simulink model "pasp_16i16c128s"  (Simulink 6.2)
settings: Solver=ode45  StartTime=0.0  StopTime=30000  RelTol=1e-3
undefined symbols (not defined in the file or in its folder): iBOB
libraries: xbsIndex_r3 x1501, casper_library x145, xps_library x90
(part 3 of 12)

== system pasp_16i16c128s/pasp/pfb_fir_real1 ==
  sync : Inport  Port=1  LatchInput=off
  pol1_in1 : Inport  Port=2  LatchInput=off
  pol1_in2 : Inport  Port=3  LatchInput=off
  pol1_in3 : Inport  Port=4  LatchInput=off
  pol1_in4 : Inport  Port=5  LatchInput=off
  pol1_in1_first_tap : Subsystem  AncestorBlock=casper_library/PFBs/first_tap_real  mask(first_tap_real){nput=0, PFBSize=5, CoeffBitWidth=8, TotalTaps=2, BitWidthIn=8, CoeffDistMem=1, CoeffRound=0, WindowType=hamming, mult_latency=2, bram_latency=2, n_inputs=2, fwidth=1}
      mask prompts: nput "This is input number:"; PFBSize "Size of PFB: (2^? pnts)"; CoeffBitWidth "Bitwidth of Coefficients:"; TotalTaps "Total Number of Taps:"; BitWidthIn "Input Bitwidth:"; CoeffDistMem "Implement Coeff Gen in Distributed Memory:"; CoeffRound "Round Coefficients?"; WindowType "Windowing Function:"; mult_latency "Mult Latency"; bram_latency "BRAM Latency"; n_inputs "Number of Simultaneous Inputs: (2^?)"; fwidth "Bit Width (normal=1)"
      mask init: same as pasp_16i16c128s/pasp/pfb_fir_real/pol1_in1_first_tap
      settings: AttributesFormatString=input=0, taps=2
      mask StyleString: edit,edit,edit,edit,edit,edit,edit,popup(bartlett|barthannwin|blackman|blackmanharris|bohamwin|chebwin|flattopwin|gausswin|hamming|hann|kaiser|nuttallwin|parzenwin|rectwin|tukeywin|triang),edit,edit,edit,edit
  pol1_in1_last_tap : Subsystem  AncestorBlock=casper_library/PFBs/last_tap_real  mask(last_tap_real){TotalTaps=2, BitWidthIn=8, BitWidthOut=18, CoeffBitWidth=8, add_latency=1, mult_latency=2, quantization=Truncate}
      mask prompts: TotalTaps "Total Number of Taps:"; BitWidthIn "Input Bitwidth:"; BitWidthOut "Output Bitwidth:"; CoeffBitWidth "Coeff Bitwidth:"; add_latency "Add Latency"; mult_latency "Mult Latency"; quantization "Quantization Behavior"
      mask init: same as pasp_16i16c128s/pasp/pfb_fir_real/pol1_in1_last_tap
      settings: AttributesFormatString=taps=2
      mask StyleString: edit,edit,edit,edit,edit,edit,popup(Truncate|Round  (unbiased: +/- Inf)|Round  (unbiased: Even Values))
  pol1_in2_first_tap : Subsystem  AncestorBlock=casper_library/PFBs/first_tap_real  mask(first_tap_real){nput=1, PFBSize=5, CoeffBitWidth=8, TotalTaps=2, BitWidthIn=8, CoeffDistMem=1, CoeffRound=0, WindowType=hamming, mult_latency=2, bram_latency=2, n_inputs=2, fwidth=1}
      mask prompts: nput "This is input number:"; PFBSize "Size of PFB: (2^? pnts)"; CoeffBitWidth "Bitwidth of Coefficients:"; TotalTaps "Total Number of Taps:"; BitWidthIn "Input Bitwidth:"; CoeffDistMem "Implement Coeff Gen in Distributed Memory:"; CoeffRound "Round Coefficients?"; WindowType "Windowing Function:"; mult_latency "Mult Latency"; bram_latency "BRAM Latency"; n_inputs "Number of Simultaneous Inputs: (2^?)"; fwidth "Bit Width (normal=1)"
      mask init: same as pasp_16i16c128s/pasp/pfb_fir_real/pol1_in1_first_tap
      settings: AttributesFormatString=input=1, taps=2
      mask StyleString: edit,edit,edit,edit,edit,edit,edit,popup(bartlett|barthannwin|blackman|blackmanharris|bohamwin|chebwin|flattopwin|gausswin|hamming|hann|kaiser|nuttallwin|parzenwin|rectwin|tukeywin|triang),edit,edit,edit,edit
  pol1_in2_last_tap : Subsystem  AncestorBlock=casper_library/PFBs/last_tap_real  mask(last_tap_real){TotalTaps=2, BitWidthIn=8, BitWidthOut=18, CoeffBitWidth=8, add_latency=1, mult_latency=2, quantization=Truncate}
      mask prompts: TotalTaps "Total Number of Taps:"; BitWidthIn "Input Bitwidth:"; BitWidthOut "Output Bitwidth:"; CoeffBitWidth "Coeff Bitwidth:"; add_latency "Add Latency"; mult_latency "Mult Latency"; quantization "Quantization Behavior"
      mask init: same as pasp_16i16c128s/pasp/pfb_fir_real/pol1_in1_last_tap
      settings: AttributesFormatString=taps=2
      mask StyleString: edit,edit,edit,edit,edit,edit,popup(Truncate|Round  (unbiased: +/- Inf)|Round  (unbiased: Even Values))
  pol1_in3_first_tap : Subsystem  AncestorBlock=casper_library/PFBs/first_tap_real  mask(first_tap_real){nput=2, PFBSize=5, CoeffBitWidth=8, TotalTaps=2, BitWidthIn=8, CoeffDistMem=1, CoeffRound=0, WindowType=hamming, mult_latency=2, bram_latency=2, n_inputs=2, fwidth=1}
      mask prompts: nput "This is input number:"; PFBSize "Size of PFB: (2^? pnts)"; CoeffBitWidth "Bitwidth of Coefficients:"; TotalTaps "Total Number of Taps:"; BitWidthIn "Input Bitwidth:"; CoeffDistMem "Implement Coeff Gen in Distributed Memory:"; CoeffRound "Round Coefficients?"; WindowType "Windowing Function:"; mult_latency "Mult Latency"; bram_latency "BRAM Latency"; n_inputs "Number of Simultaneous Inputs: (2^?)"; fwidth "Bit Width (normal=1)"
      mask init: same as pasp_16i16c128s/pasp/pfb_fir_real/pol1_in1_first_tap
      settings: AttributesFormatString=input=2, taps=2
      mask StyleString: edit,edit,edit,edit,edit,edit,edit,popup(bartlett|barthannwin|blackman|blackmanharris|bohamwin|chebwin|flattopwin|gausswin|hamming|hann|kaiser|nuttallwin|parzenwin|rectwin|tukeywin|triang),edit,edit,edit,edit
  pol1_in3_last_tap : Subsystem  AncestorBlock=casper_library/PFBs/last_tap_real  mask(last_tap_real){TotalTaps=2, BitWidthIn=8, BitWidthOut=18, CoeffBitWidth=8, add_latency=1, mult_latency=2, quantization=Truncate}
      mask prompts: TotalTaps "Total Number of Taps:"; BitWidthIn "Input Bitwidth:"; BitWidthOut "Output Bitwidth:"; CoeffBitWidth "Coeff Bitwidth:"; add_latency "Add Latency"; mult_latency "Mult Latency"; quantization "Quantization Behavior"
      mask init: same as pasp_16i16c128s/pasp/pfb_fir_real/pol1_in1_last_tap
      settings: AttributesFormatString=taps=2
      mask StyleString: edit,edit,edit,edit,edit,edit,popup(Truncate|Round  (unbiased: +/- Inf)|Round  (unbiased: Even Values))
  pol1_in4_first_tap : Subsystem  AncestorBlock=casper_library/PFBs/first_tap_real  mask(first_tap_real){nput=3, PFBSize=5, CoeffBitWidth=8, TotalTaps=2, BitWidthIn=8, CoeffDistMem=1, CoeffRound=0, WindowType=hamming, mult_latency=2, bram_latency=2, n_inputs=2, fwidth=1}
      mask prompts: nput "This is input number:"; PFBSize "Size of PFB: (2^? pnts)"; CoeffBitWidth "Bitwidth of Coefficients:"; TotalTaps "Total Number of Taps:"; BitWidthIn "Input Bitwidth:"; CoeffDistMem "Implement Coeff Gen in Distributed Memory:"; CoeffRound "Round Coefficients?"; WindowType "Windowing Function:"; mult_latency "Mult Latency"; bram_latency "BRAM Latency"; n_inputs "Number of Simultaneous Inputs: (2^?)"; fwidth "Bit Width (normal=1)"
      mask init: same as pasp_16i16c128s/pasp/pfb_fir_real/pol1_in1_first_tap
      settings: AttributesFormatString=input=3, taps=2
      mask StyleString: edit,edit,edit,edit,edit,edit,edit,popup(bartlett|barthannwin|blackman|blackmanharris|bohamwin|chebwin|flattopwin|gausswin|hamming|hann|kaiser|nuttallwin|parzenwin|rectwin|tukeywin|triang),edit,edit,edit,edit
  pol1_in4_last_tap : Subsystem  AncestorBlock=casper_library/PFBs/last_tap_real  mask(last_tap_real){TotalTaps=2, BitWidthIn=8, BitWidthOut=18, CoeffBitWidth=8, add_latency=1, mult_latency=2, quantization=Truncate}
      mask prompts: TotalTaps "Total Number of Taps:"; BitWidthIn "Input Bitwidth:"; BitWidthOut "Output Bitwidth:"; CoeffBitWidth "Coeff Bitwidth:"; add_latency "Add Latency"; mult_latency "Mult Latency"; quantization "Quantization Behavior"
      mask init: same as pasp_16i16c128s/pasp/pfb_fir_real/pol1_in1_last_tap
      settings: AttributesFormatString=taps=2
      mask StyleString: edit,edit,edit,edit,edit,edit,popup(Truncate|Round  (unbiased: +/- Inf)|Round  (unbiased: Even Values))
  sync_out : Outport
  pol1_out1 : Outport  Port=2
  pol1_out2 : Outport  Port=3
  pol1_out3 : Outport  Port=4
  pol1_out4 : Outport  Port=5
  wires:
  pol1_in1/1 -> pol1_in1_first_tap/1(din)
  sync/1 -> pol1_in1_first_tap/2(sync), pol1_in2_first_tap/2(sync), pol1_in3_first_tap/2(sync), pol1_in4_first_tap/2(sync)
  pol1_in1_first_tap/1(dout) -> pol1_in1_last_tap/1(din)
  pol1_in1_first_tap/2(sync_out) -> pol1_in1_last_tap/2(sync)
  pol1_in1_first_tap/3(coeff_out) -> pol1_in1_last_tap/3(coeff)
  pol1_in1_first_tap/4(taps_out) -> pol1_in1_last_tap/4(taps)
  pol1_in1_last_tap/1(dout) -> pol1_out1/1
  pol1_in1_last_tap/2(sync_out) -> sync_out/1
  pol1_in2/1 -> pol1_in2_first_tap/1(din)
  pol1_in2_first_tap/1(dout) -> pol1_in2_last_tap/1(din)
  pol1_in2_first_tap/2(sync_out) -> pol1_in2_last_tap/2(sync)
  pol1_in2_first_tap/3(coeff_out) -> pol1_in2_last_tap/3(coeff)
  pol1_in2_first_tap/4(taps_out) -> pol1_in2_last_tap/4(taps)
  pol1_in2_last_tap/1(dout) -> pol1_out2/1
  pol1_in3/1 -> pol1_in3_first_tap/1(din)
  pol1_in3_first_tap/1(dout) -> pol1_in3_last_tap/1(din)
  pol1_in3_first_tap/2(sync_out) -> pol1_in3_last_tap/2(sync)
  pol1_in3_first_tap/3(coeff_out) -> pol1_in3_last_tap/3(coeff)
  pol1_in3_first_tap/4(taps_out) -> pol1_in3_last_tap/4(taps)
  pol1_in3_last_tap/1(dout) -> pol1_out3/1
  pol1_in4/1 -> pol1_in4_first_tap/1(din)
  pol1_in4_first_tap/1(dout) -> pol1_in4_last_tap/1(din)
  pol1_in4_first_tap/2(sync_out) -> pol1_in4_last_tap/2(sync)
  pol1_in4_first_tap/3(coeff_out) -> pol1_in4_last_tap/3(coeff)
  pol1_in4_first_tap/4(taps_out) -> pol1_in4_last_tap/4(taps)
  pol1_in4_last_tap/1(dout) -> pol1_out4/1

== system pasp_16i16c128s/pasp/reorder ==
  sync : Inport  Port=1  LatchInput=off
  en : Inport  Port=2  LatchInput=off
  din0 : Inport  Port=3  LatchInput=off
  din1 : Inport  Port=4  LatchInput=off
  Counter : xbsIndex_r3/Counter  cnt_type=Count Limited  n_bits=6  bin_pt=0  arith_type=Unsigned  start_count=0  cnt_to=63  cnt_by_val=1  operation=Up  explicit_period=off  period=1  load_pin=off  rst=on  en=on  dbl_ovrd=off  show_param=off  use_rpm=on  gen_core=off
      settings: xl_area=[0, 0, 0, 0, 0, 0, 0]
  Mux : xbsIndex_r3/Mux  inputs=4  precision=Full  arith_type="Signed  (2's comp)"  n_bits=8  bin_pt=2  quantization=Truncate  overflow=Wrap  latency=1  explicit_period=off  period=1  en=off  dbl_ovrd=off  show_param=off  mux_type=off  use_rpm=off  gen_core=off
      settings: xl_area=[0, 0, 0, 0, 0, 0, 0]
  Slice1 : xbsIndex_r3/Slice  mode=Upper Bit Location + Width  nbits=2  bit1=0  base1=MSB of Input  bit0=0  base0=LSB of Input  boolean_output=off  explicit_period=off  period=1  dbl_ovrd=off
  Slice2 : xbsIndex_r3/Slice  mode=Lower Bit Location + Width  nbits=4  bit1=0  base1=MSB of Input  bit0=0  base0=LSB of Input  boolean_output=off  explicit_period=off  period=1  dbl_ovrd=off
  bram0 : xbsIndex_r3/Single Port RAM  depth=16  initVector=sin(pi*(0:15)/16)  write_mode=Read Before Write  latency=2  init_zero=on  explicit_period=off  period=1  rst=off  init_reg=0  en=off  dbl_ovrd=off  show_param=off  distributed_mem=off  use_rpm=off  gen_core=off
      settings: xl_area=[0, 0, 0, 0, 0, 0, 0]
  bram1 : xbsIndex_r3/Single Port RAM  depth=16  initVector=sin(pi*(0:15)/16)  write_mode=Read Before Write  latency=2  init_zero=on  explicit_period=off  period=1  rst=off  init_reg=0  en=off  dbl_ovrd=off  show_param=off  distributed_mem=off  use_rpm=off  gen_core=off
      settings: xl_area=[0, 0, 0, 0, 0, 0, 0]
  delay_d0 : xbsIndex_r3/Delay  latency=3  reg_retiming=off  explicit_period=off  period=1  en=off  accept_only_valid=off  init_zero=on  dbl_ovrd=off  show_param=off
      settings: xl_area=[0, 0, 0, 0, 0, 0, 0]
  delay_din0 : xbsIndex_r3/Delay  latency=4  reg_retiming=off  explicit_period=off  period=1  en=off  accept_only_valid=off  init_zero=on  dbl_ovrd=off  show_param=off
      settings: xl_area=[0, 0, 0, 0, 0, 0, 0]
  delay_din1 : xbsIndex_r3/Delay  latency=4  reg_retiming=off  explicit_period=off  period=1  en=off  accept_only_valid=off  init_zero=on  dbl_ovrd=off  show_param=off
      settings: xl_area=[0, 0, 0, 0, 0, 0, 0]
  delay_map1 : xbsIndex_r3/Delay  latency=2*map_latency  reg_retiming=off  explicit_period=off  period=1  en=off  accept_only_valid=off  init_zero=on  dbl_ovrd=off  show_param=off
      settings: xl_area=[0, 0, 0, 0, 0, 0, 0]
  delay_map2 : xbsIndex_r3/Delay  latency=1*map_latency  reg_retiming=off  explicit_period=off  period=1  en=off  accept_only_valid=off  init_zero=on  dbl_ovrd=off  show_param=off
      settings: xl_area=[0, 0, 0, 0, 0, 0, 0]
  delay_map3 : xbsIndex_r3/Delay  latency=0*map_latency  reg_retiming=off  explicit_period=off  period=1  en=off  accept_only_valid=off  init_zero=on  dbl_ovrd=off  show_param=off
      settings: xl_area=[0, 0, 0, 0, 0, 0, 0]
  delay_sel : xbsIndex_r3/Delay  latency=3  reg_retiming=off  explicit_period=off  period=1  en=off  accept_only_valid=off  init_zero=on  dbl_ovrd=off  show_param=off
      settings: xl_area=[0, 0, 0, 0, 0, 0, 0]
  delay_valid : xbsIndex_r3/Delay  latency=3  reg_retiming=off  explicit_period=off  period=1  en=off  accept_only_valid=off  init_zero=on  dbl_ovrd=off  show_param=off
      settings: xl_area=[0, 0, 0, 0, 0, 0, 0]
  delay_we : xbsIndex_r3/Delay  latency=3  reg_retiming=off  explicit_period=off  period=1  en=off  accept_only_valid=off  init_zero=on  dbl_ovrd=off  show_param=off
      settings: xl_area=[0, 0, 0, 0, 0, 0, 0]
  map1 : xbsIndex_r3/ROM  depth=16  initVector=[0 8 1 9 2 10 3 11 4 12 5 13 6 14 7 15]  arith_type=Unsigned  n_bits=4  bin_pt=0  latency=1  init_zero=on  explicit_period=off  period=1  rst=off  init_reg=0  en=off  dbl_ovrd=off  show_param=on  distributed_mem=off  use_rpm=off  gen_core=off
      settings: xl_area=[0, 0, 0, 0, 0, 0, 0]
  map2 : xbsIndex_r3/ROM  depth=16  initVector=[0 8 1 9 2 10 3 11 4 12 5 13 6 14 7 15]  arith_type=Unsigned  n_bits=4  bin_pt=0  latency=1  init_zero=on  explicit_period=off  period=1  rst=off  init_reg=0  en=off  dbl_ovrd=off  show_param=on  distributed_mem=off  use_rpm=off  gen_core=off
      settings: xl_area=[0, 0, 0, 0, 0, 0, 0]
  map3 : xbsIndex_r3/ROM  depth=16  initVector=[0 8 1 9 2 10 3 11 4 12 5 13 6 14 7 15]  arith_type=Unsigned  n_bits=4  bin_pt=0  latency=1  init_zero=on  explicit_period=off  period=1  rst=off  init_reg=0  en=off  dbl_ovrd=off  show_param=on  distributed_mem=off  use_rpm=off  gen_core=off
      settings: xl_area=[0, 0, 0, 0, 0, 0, 0]
  post_sync_delay : xbsIndex_r3/Delay  latency=3  reg_retiming=off  explicit_period=off  period=1  en=off  accept_only_valid=off  init_zero=on  dbl_ovrd=off  show_param=off
      settings: xl_area=[0, 0, 0, 0, 0, 0, 0]
  pre_sync_delay : xbsIndex_r3/Delay  latency=3  reg_retiming=off  explicit_period=off  period=1  en=off  accept_only_valid=off  init_zero=on  dbl_ovrd=off  show_param=off
      settings: xl_area=[0, 0, 0, 0, 0, 0, 0]
  sync_delay_en : casper_library/Delays/sync_delay_en  DelayLen=16
      link override Constant: equ=P=C
      link override Constant1: equ=P=C
      link override Constant2: equ=P=C
      link override Constant3: equ=P=C
  sync_out : Outport
  valid : Outport  Port=2
  dout0 : Outport  Port=3
  dout1 : Outport  Port=4
  wires:
  sync/1 -> Counter/1, pre_sync_delay/1
  en/1 -> Counter/2, sync_delay_en/2, delay_we/1
  Counter/1 -> Slice1/1, Slice2/1
  Slice1/1 -> delay_sel/1
  delay_sel/1 -> Mux/1
  Slice2/1 -> delay_d0/1, map1/1
  delay_d0/1 -> Mux/2
  pre_sync_delay/1 -> sync_delay_en/1
  sync_delay_en/1 -> post_sync_delay/1
  post_sync_delay/1 -> sync_out/1
  delay_we/1 -> delay_valid/1, bram0/3, bram1/3
  delay_valid/1 -> valid/1
  Mux/1 -> bram0/1, bram1/1
  din0/1 -> delay_din0/1
  delay_din0/1 -> bram0/2
  bram0/1 -> dout0/1
  din1/1 -> delay_din1/1
  delay_din1/1 -> bram1/2
  bram1/1 -> dout1/1
  map1/1 -> delay_map1/1, map2/1
  delay_map1/1 -> Mux/3
  map2/1 -> delay_map2/1, map3/1
  delay_map2/1 -> Mux/4
  map3/1 -> delay_map3/1
  delay_map3/1 -> Mux/5

== system pasp_16i16c128s/pasp/scale1 ==
  note: Unsigned, 18-bits, b.p. at 12
  note: Output complex signed R/I 18-bits, b.p. at 17
  note: Input complex signed R/I 18-bits, b.p. at 17
  coeff : Inport  Orientation=down  Port=1  LatchInput=off
  data_in : Inport  Port=2  LatchInput=off
  c_to_ri : casper_library/Misc/c_to_ri  n_bits=18  bin_pt=17
      settings: AttributesFormatString=18_17 r/i
  mult_coeff_fft_imag : xbsIndex_r3/Mult  precision=User Defined  arith_type="Signed  (2's comp)"  n_bits=18  bin_pt=17  quantization=Truncate  overflow=Saturate  latency=6  explicit_period=off  period=1  en=off  dbl_ovrd=off  show_param=on  mult_type=Parallel  oversample=2  use_embedded=on  pipeline=on  use_rpm=on  placement_style=Rectangular Shape  gen_core=off
      settings: xl_area=[0, 0, 0, 0, 0, 0, 0]
  mult_coeff_fft_real : xbsIndex_r3/Mult  precision=User Defined  arith_type="Signed  (2's comp)"  n_bits=18  bin_pt=17  quantization=Truncate  overflow=Saturate  latency=6  explicit_period=off  period=1  en=off  dbl_ovrd=off  show_param=on  mult_type=Parallel  oversample=2  use_embedded=on  pipeline=on  use_rpm=on  placement_style=Rectangular Shape  gen_core=off
      settings: xl_area=[0, 0, 0, 0, 0, 0, 0]
  ri_to_c : casper_library/Misc/ri_to_c
  data_out : Outport
  wires:
  c_to_ri/1 -> mult_coeff_fft_real/2
  c_to_ri/2 -> mult_coeff_fft_imag/2
  mult_coeff_fft_real/1 -> ri_to_c/1
  mult_coeff_fft_imag/1 -> ri_to_c/2
  coeff/1 -> mult_coeff_fft_real/1, mult_coeff_fft_imag/1
  ri_to_c/1 -> data_out/1
  data_in/1 -> c_to_ri/1

== system pasp_16i16c128s/pasp/scale2 ==
  note: Input complex signed R/I 18-bits, b.p. at 17
  note: Output complex signed R/I 18-bits, b.p. at 17
  note: Unsigned, 18-bits, b.p. at 12
  coeff : Inport  Orientation=down  Port=1  LatchInput=off
  data_in : Inport  Port=2  LatchInput=off
  c_to_ri : casper_library/Misc/c_to_ri  n_bits=18  bin_pt=17
      settings: AttributesFormatString=18_17 r/i
  mult_coeff_fft_imag : xbsIndex_r3/Mult  precision=User Defined  arith_type="Signed  (2's comp)"  n_bits=18  bin_pt=17  quantization=Truncate  overflow=Saturate  latency=6  explicit_period=off  period=1  en=off  dbl_ovrd=off  show_param=on  mult_type=Parallel  oversample=2  use_embedded=on  pipeline=on  use_rpm=on  placement_style=Rectangular Shape  gen_core=off
      settings: xl_area=[0, 0, 0, 0, 0, 0, 0]
  mult_coeff_fft_real : xbsIndex_r3/Mult  precision=User Defined  arith_type="Signed  (2's comp)"  n_bits=18  bin_pt=17  quantization=Truncate  overflow=Saturate  latency=6  explicit_period=off  period=1  en=off  dbl_ovrd=off  show_param=on  mult_type=Parallel  oversample=2  use_embedded=on  pipeline=on  use_rpm=on  placement_style=Rectangular Shape  gen_core=off
      settings: xl_area=[0, 0, 0, 0, 0, 0, 0]
  ri_to_c : casper_library/Misc/ri_to_c
  data_out : Outport
  wires:
  data_in/1 -> c_to_ri/1
  ri_to_c/1 -> data_out/1
  coeff/1 -> mult_coeff_fft_imag/1, mult_coeff_fft_real/1
  mult_coeff_fft_imag/1 -> ri_to_c/2
  mult_coeff_fft_real/1 -> ri_to_c/1
  c_to_ri/2 -> mult_coeff_fft_imag/2
  c_to_ri/1 -> mult_coeff_fft_real/2

== system pasp_16i16c128s/pasp/scale3 ==
  note: Unsigned, 18-bits, b.p. at 12
  note: Output complex signed R/I 18-bits, b.p. at 17
  note: Input complex signed R/I 18-bits, b.p. at 17
  coeff : Inport  Orientation=down  Port=1  LatchInput=off
  data_in : Inport  Port=2  LatchInput=off
  c_to_ri : casper_library/Misc/c_to_ri  n_bits=18  bin_pt=17
      settings: AttributesFormatString=18_17 r/i
  mult_coeff_fft_imag : xbsIndex_r3/Mult  precision=User Defined  arith_type="Signed  (2's comp)"  n_bits=18  bin_pt=17  quantization=Truncate  overflow=Saturate  latency=6  explicit_period=off  period=1  en=off  dbl_ovrd=off  show_param=on  mult_type=Parallel  oversample=2  use_embedded=on  pipeline=on  use_rpm=on  placement_style=Rectangular Shape  gen_core=off
      settings: xl_area=[0, 0, 0, 0, 0, 0, 0]
  mult_coeff_fft_real : xbsIndex_r3/Mult  precision=User Defined  arith_type="Signed  (2's comp)"  n_bits=18  bin_pt=17  quantization=Truncate  overflow=Saturate  latency=6  explicit_period=off  period=1  en=off  dbl_ovrd=off  show_param=on  mult_type=Parallel  oversample=2  use_embedded=on  pipeline=on  use_rpm=on  placement_style=Rectangular Shape  gen_core=off
      settings: xl_area=[0, 0, 0, 0, 0, 0, 0]
  ri_to_c : casper_library/Misc/ri_to_c
  data_out : Outport
  wires:
  c_to_ri/1 -> mult_coeff_fft_real/2
  c_to_ri/2 -> mult_coeff_fft_imag/2
  mult_coeff_fft_real/1 -> ri_to_c/1
  mult_coeff_fft_imag/1 -> ri_to_c/2
  coeff/1 -> mult_coeff_fft_real/1, mult_coeff_fft_imag/1
  ri_to_c/1 -> data_out/1
  data_in/1 -> c_to_ri/1

== system pasp_16i16c128s/pasp/scale4 ==
  note: Input complex signed R/I 18-bits, b.p. at 17
  note: Output complex signed R/I 18-bits, b.p. at 17
  note: Unsigned, 18-bits, b.p. at 12
  coeff : Inport  Orientation=down  Port=1  LatchInput=off
  data_in : Inport  Port=2  LatchInput=off
  c_to_ri : casper_library/Misc/c_to_ri  n_bits=18  bin_pt=17
      settings: AttributesFormatString=18_17 r/i
  mult_coeff_fft_imag : xbsIndex_r3/Mult  precision=User Defined  arith_type="Signed  (2's comp)"  n_bits=18  bin_pt=17  quantization=Truncate  overflow=Saturate  latency=6  explicit_period=off  period=1  en=off  dbl_ovrd=off  show_param=on  mult_type=Parallel  oversample=2  use_embedded=on  pipeline=on  use_rpm=on  placement_style=Rectangular Shape  gen_core=off
      settings: xl_area=[0, 0, 0, 0, 0, 0, 0]
  mult_coeff_fft_real : xbsIndex_r3/Mult  precision=User Defined  arith_type="Signed  (2's comp)"  n_bits=18  bin_pt=17  quantization=Truncate  overflow=Saturate  latency=6  explicit_period=off  period=1  en=off  dbl_ovrd=off  show_param=on  mult_type=Parallel  oversample=2  use_embedded=on  pipeline=on  use_rpm=on  placement_style=Rectangular Shape  gen_core=off
      settings: xl_area=[0, 0, 0, 0, 0, 0, 0]
  ri_to_c : casper_library/Misc/ri_to_c
  data_out : Outport
  wires:
  data_in/1 -> c_to_ri/1
  ri_to_c/1 -> data_out/1
  coeff/1 -> mult_coeff_fft_imag/1, mult_coeff_fft_real/1
  mult_coeff_fft_imag/1 -> ri_to_c/2
  mult_coeff_fft_real/1 -> ri_to_c/1
  c_to_ri/2 -> mult_coeff_fft_imag/2
  c_to_ri/1 -> mult_coeff_fft_real/2

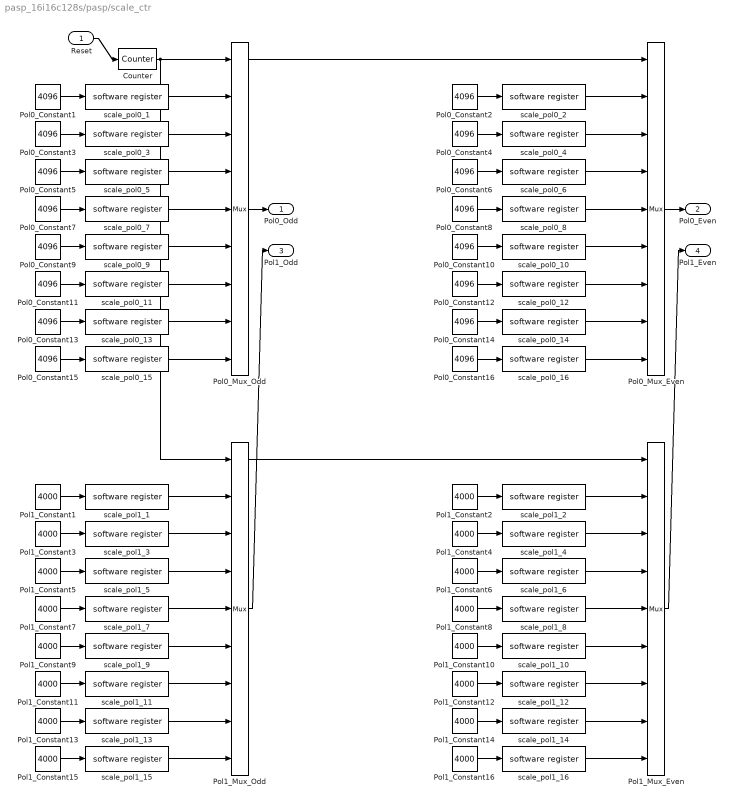
== system pasp_16i16c128s/pasp/scale_ctr ==
  Reset : Inport  Port=1  LatchInput=off
  Counter : xbsIndex_r3/Counter  cnt_type=Free Running  n_bits=3  bin_pt=0  arith_type=Unsigned  start_count=0  cnt_to=Inf  cnt_by_val=1  operation=Up  explicit_period=off  period=1  load_pin=off  rst=on  en=off  dbl_ovrd=off  show_param=off  use_rpm=on  gen_core=off
      settings: xl_area=[0, 0, 0, 0, 0, 0, 0]
  Pol0_Constant{1..16} (16 alike) : Constant  Value=4096
  Pol0_Mux_Even : xbsIndex_r3/Mux  inputs=8  precision=Full  arith_type="Signed  (2's comp)"  n_bits=8  bin_pt=2  quantization=Truncate  overflow=Wrap  latency=3  explicit_period=off  period=1  en=off  dbl_ovrd=off  show_param=off  mux_type=off  use_rpm=off  gen_core=off
      settings: xl_area=[0, 0, 0, 0, 0, 0, 0]
  Pol0_Mux_Odd : xbsIndex_r3/Mux  inputs=8  precision=Full  arith_type="Signed  (2's comp)"  n_bits=8  bin_pt=2  quantization=Truncate  overflow=Wrap  latency=3  explicit_period=off  period=1  en=off  dbl_ovrd=off  show_param=off  mux_type=off  use_rpm=off  gen_core=off
      settings: xl_area=[0, 0, 0, 0, 0, 0, 0]
  Pol1_Constant{1..16} (16 alike) : Constant  Value=4000
  Pol1_Mux_Even : xbsIndex_r3/Mux  inputs=8  precision=Full  arith_type="Signed  (2's comp)"  n_bits=8  bin_pt=2  quantization=Truncate  overflow=Wrap  latency=3  explicit_period=off  period=1  en=off  dbl_ovrd=off  show_param=off  mux_type=off  use_rpm=off  gen_core=off
      settings: xl_area=[0, 0, 0, 0, 0, 0, 0]
  Pol1_Mux_Odd : xbsIndex_r3/Mux  inputs=8  precision=Full  arith_type="Signed  (2's comp)"  n_bits=8  bin_pt=2  quantization=Truncate  overflow=Wrap  latency=3  explicit_period=off  period=1  en=off  dbl_ovrd=off  show_param=off  mux_type=off  use_rpm=off  gen_core=off
      settings: xl_area=[0, 0, 0, 0, 0, 0, 0]
  scale_pol0_1 : xps_library/software register  Tag=xps:sw_reg  io_dir=From Processor  arith_type=Unsigned  bitwidth=32  bin_pt=0  sample_period=1  gw_name=pasp_16i16c128s_pasp_scale_ctr_scale_pol0_1_user_data_out
  scale_pol0_10 : xps_library/software register  Tag=xps:sw_reg  io_dir=From Processor  arith_type=Unsigned  bitwidth=32  bin_pt=0  sample_period=1  gw_name=pasp_16i16c128s_pasp_scale_ctr_scale_pol0_10_user_data_out
  scale_pol0_11 : xps_library/software register  Tag=xps:sw_reg  io_dir=From Processor  arith_type=Unsigned  bitwidth=32  bin_pt=0  sample_period=1  gw_name=pasp_16i16c128s_pasp_scale_ctr_scale_pol0_11_user_data_out
  scale_pol0_12 : xps_library/software register  Tag=xps:sw_reg  io_dir=From Processor  arith_type=Unsigned  bitwidth=32  bin_pt=0  sample_period=1  gw_name=pasp_16i16c128s_pasp_scale_ctr_scale_pol0_12_user_data_out
  scale_pol0_13 : xps_library/software register  Tag=xps:sw_reg  io_dir=From Processor  arith_type=Unsigned  bitwidth=32  bin_pt=0  sample_period=1  gw_name=pasp_16i16c128s_pasp_scale_ctr_scale_pol0_13_user_data_out
  scale_pol0_14 : xps_library/software register  Tag=xps:sw_reg  io_dir=From Processor  arith_type=Unsigned  bitwidth=32  bin_pt=0  sample_period=1  gw_name=pasp_16i16c128s_pasp_scale_ctr_scale_pol0_14_user_data_out
  scale_pol0_15 : xps_library/software register  Tag=xps:sw_reg  io_dir=From Processor  arith_type=Unsigned  bitwidth=32  bin_pt=0  sample_period=1  gw_name=pasp_16i16c128s_pasp_scale_ctr_scale_pol0_15_user_data_out
  scale_pol0_16 : xps_library/software register  Tag=xps:sw_reg  io_dir=From Processor  arith_type=Unsigned  bitwidth=32  bin_pt=0  sample_period=1  gw_name=pasp_16i16c128s_pasp_scale_ctr_scale_pol0_16_user_data_out
  scale_pol0_2 : xps_library/software register  Tag=xps:sw_reg  io_dir=From Processor  arith_type=Unsigned  bitwidth=32  bin_pt=0  sample_period=1  gw_name=pasp_16i16c128s_pasp_scale_ctr_scale_pol0_2_user_data_out
  scale_pol0_3 : xps_library/software register  Tag=xps:sw_reg  io_dir=From Processor  arith_type=Unsigned  bitwidth=32  bin_pt=0  sample_period=1  gw_name=pasp_16i16c128s_pasp_scale_ctr_scale_pol0_3_user_data_out
  scale_pol0_4 : xps_library/software register  Tag=xps:sw_reg  io_dir=From Processor  arith_type=Unsigned  bitwidth=32  bin_pt=0  sample_period=1  gw_name=pasp_16i16c128s_pasp_scale_ctr_scale_pol0_4_user_data_out
  scale_pol0_5 : xps_library/software register  Tag=xps:sw_reg  io_dir=From Processor  arith_type=Unsigned  bitwidth=32  bin_pt=0  sample_period=1  gw_name=pasp_16i16c128s_pasp_scale_ctr_scale_pol0_5_user_data_out
  scale_pol0_6 : xps_library/software register  Tag=xps:sw_reg  io_dir=From Processor  arith_type=Unsigned  bitwidth=32  bin_pt=0  sample_period=1  gw_name=pasp_16i16c128s_pasp_scale_ctr_scale_pol0_6_user_data_out
  scale_pol0_7 : xps_library/software register  Tag=xps:sw_reg  io_dir=From Processor  arith_type=Unsigned  bitwidth=32  bin_pt=0  sample_period=1  gw_name=pasp_16i16c128s_pasp_scale_ctr_scale_pol0_7_user_data_out
  scale_pol0_8 : xps_library/software register  Tag=xps:sw_reg  io_dir=From Processor  arith_type=Unsigned  bitwidth=32  bin_pt=0  sample_period=1  gw_name=pasp_16i16c128s_pasp_scale_ctr_scale_pol0_8_user_data_out
  scale_pol0_9 : xps_library/software register  Tag=xps:sw_reg  io_dir=From Processor  arith_type=Unsigned  bitwidth=32  bin_pt=0  sample_period=1  gw_name=pasp_16i16c128s_pasp_scale_ctr_scale_pol0_9_user_data_out
  scale_pol1_1 : xps_library/software register  Tag=xps:sw_reg  io_dir=From Processor  arith_type=Unsigned  bitwidth=32  bin_pt=0  sample_period=1  gw_name=pasp_16i16c128s_pasp_scale_ctr_scale_pol1_1_user_data_out
  scale_pol1_10 : xps_library/software register  Tag=xps:sw_reg  io_dir=From Processor  arith_type=Unsigned  bitwidth=32  bin_pt=0  sample_period=1  gw_name=pasp_16i16c128s_pasp_scale_ctr_scale_pol1_10_user_data_out
  scale_pol1_11 : xps_library/software register  Tag=xps:sw_reg  io_dir=From Processor  arith_type=Unsigned  bitwidth=32  bin_pt=0  sample_period=1  gw_name=pasp_16i16c128s_pasp_scale_ctr_scale_pol1_11_user_data_out
  scale_pol1_12 : xps_library/software register  Tag=xps:sw_reg  io_dir=From Processor  arith_type=Unsigned  bitwidth=32  bin_pt=0  sample_period=1  gw_name=pasp_16i16c128s_pasp_scale_ctr_scale_pol1_12_user_data_out
  scale_pol1_13 : xps_library/software register  Tag=xps:sw_reg  io_dir=From Processor  arith_type=Unsigned  bitwidth=32  bin_pt=0  sample_period=1  gw_name=pasp_16i16c128s_pasp_scale_ctr_scale_pol1_13_user_data_out
  scale_pol1_14 : xps_library/software register  Tag=xps:sw_reg  io_dir=From Processor  arith_type=Unsigned  bitwidth=32  bin_pt=0  sample_period=1  gw_name=pasp_16i16c128s_pasp_scale_ctr_scale_pol1_14_user_data_out
  scale_pol1_15 : xps_library/software register  Tag=xps:sw_reg  io_dir=From Processor  arith_type=Unsigned  bitwidth=32  bin_pt=0  sample_period=1  gw_name=pasp_16i16c128s_pasp_scale_ctr_scale_pol1_15_user_data_out
  scale_pol1_16 : xps_library/software register  Tag=xps:sw_reg  io_dir=From Processor  arith_type=Unsigned  bitwidth=32  bin_pt=0  sample_period=1  gw_name=pasp_16i16c128s_pasp_scale_ctr_scale_pol1_16_user_data_out
  scale_pol1_2 : xps_library/software register  Tag=xps:sw_reg  io_dir=From Processor  arith_type=Unsigned  bitwidth=32  bin_pt=0  sample_period=1  gw_name=pasp_16i16c128s_pasp_scale_ctr_scale_pol1_2_user_data_out
  scale_pol1_3 : xps_library/software register  Tag=xps:sw_reg  io_dir=From Processor  arith_type=Unsigned  bitwidth=32  bin_pt=0  sample_period=1  gw_name=pasp_16i16c128s_pasp_scale_ctr_scale_pol1_3_user_data_out
  scale_pol1_4 : xps_library/software register  Tag=xps:sw_reg  io_dir=From Processor  arith_type=Unsigned  bitwidth=32  bin_pt=0  sample_period=1  gw_name=pasp_16i16c128s_pasp_scale_ctr_scale_pol1_4_user_data_out
  scale_pol1_5 : xps_library/software register  Tag=xps:sw_reg  io_dir=From Processor  arith_type=Unsigned  bitwidth=32  bin_pt=0  sample_period=1  gw_name=pasp_16i16c128s_pasp_scale_ctr_scale_pol1_5_user_data_out
  scale_pol1_6 : xps_library/software register  Tag=xps:sw_reg  io_dir=From Processor  arith_type=Unsigned  bitwidth=32  bin_pt=0  sample_period=1  gw_name=pasp_16i16c128s_pasp_scale_ctr_scale_pol1_6_user_data_out
  scale_pol1_7 : xps_library/software register  Tag=xps:sw_reg  io_dir=From Processor  arith_type=Unsigned  bitwidth=32  bin_pt=0  sample_period=1  gw_name=pasp_16i16c128s_pasp_scale_ctr_scale_pol1_7_user_data_out
  scale_pol1_8 : xps_library/software register  Tag=xps:sw_reg  io_dir=From Processor  arith_type=Unsigned  bitwidth=32  bin_pt=0  sample_period=1  gw_name=pasp_16i16c128s_pasp_scale_ctr_scale_pol1_8_user_data_out
  scale_pol1_9 : xps_library/software register  Tag=xps:sw_reg  io_dir=From Processor  arith_type=Unsigned  bitwidth=32  bin_pt=0  sample_period=1  gw_name=pasp_16i16c128s_pasp_scale_ctr_scale_pol1_9_user_data_out
  Pol0_Odd : Outport
  Pol0_Even : Outport  Port=2
  Pol1_Odd : Outport  Port=3
  Pol1_Even : Outport  Port=4
  wires:
  Reset/1 -> Counter/1
  Counter/1 -> Pol0_Mux_Odd/1, Pol1_Mux_Odd/1, Pol0_Mux_Even/1, Pol1_Mux_Even/1
  Pol0_Mux_Odd/1 -> Pol0_Odd/1
  Pol1_Mux_Odd/1 -> Pol1_Odd/1
  Pol0_Mux_Even/1 -> Pol0_Even/1
  Pol1_Mux_Even/1 -> Pol1_Even/1
  Pol0_Constant1/1 -> scale_pol0_1/1
  scale_pol0_1/1 -> Pol0_Mux_Odd/2
  Pol1_Constant1/1 -> scale_pol1_1/1
  scale_pol1_1/1 -> Pol1_Mux_Odd/2
  Pol0_Constant3/1 -> scale_pol0_3/1
  scale_pol0_3/1 -> Pol0_Mux_Odd/3
  Pol1_Constant3/1 -> scale_pol1_3/1
  scale_pol1_3/1 -> Pol1_Mux_Odd/3
  Pol0_Constant5/1 -> scale_pol0_5/1
  scale_pol0_5/1 -> Pol0_Mux_Odd/4
  Pol1_Constant5/1 -> scale_pol1_5/1
  scale_pol1_5/1 -> Pol1_Mux_Odd/4
  Pol0_Constant7/1 -> scale_pol0_7/1
  scale_pol0_7/1 -> Pol0_Mux_Odd/5
  Pol1_Constant7/1 -> scale_pol1_7/1
  scale_pol1_7/1 -> Pol1_Mux_Odd/5
  Pol0_Constant9/1 -> scale_pol0_9/1
  scale_pol0_9/1 -> Pol0_Mux_Odd/6
  Pol1_Constant9/1 -> scale_pol1_9/1
  scale_pol1_9/1 -> Pol1_Mux_Odd/6
  Pol0_Constant11/1 -> scale_pol0_11/1
  scale_pol0_11/1 -> Pol0_Mux_Odd/7
  Pol1_Constant11/1 -> scale_pol1_11/1
  scale_pol1_11/1 -> Pol1_Mux_Odd/7
  Pol0_Constant13/1 -> scale_pol0_13/1
  scale_pol0_13/1 -> Pol0_Mux_Odd/8
  Pol1_Constant13/1 -> scale_pol1_13/1
  scale_pol1_13/1 -> Pol1_Mux_Odd/8
  Pol0_Constant15/1 -> scale_pol0_15/1
  scale_pol0_15/1 -> Pol0_Mux_Odd/9
  Pol1_Constant15/1 -> scale_pol1_15/1
  scale_pol1_15/1 -> Pol1_Mux_Odd/9
  Pol0_Constant2/1 -> scale_pol0_2/1
  scale_pol0_2/1 -> Pol0_Mux_Even/2
  Pol1_Constant2/1 -> scale_pol1_2/1
  scale_pol1_2/1 -> Pol1_Mux_Even/2
  Pol0_Constant4/1 -> scale_pol0_4/1
  scale_pol0_4/1 -> Pol0_Mux_Even/3
  Pol1_Constant4/1 -> scale_pol1_4/1
  scale_pol1_4/1 -> Pol1_Mux_Even/3
  Pol0_Constant6/1 -> scale_pol0_6/1
  scale_pol0_6/1 -> Pol0_Mux_Even/4
  Pol1_Constant6/1 -> scale_pol1_6/1
  scale_pol1_6/1 -> Pol1_Mux_Even/4
  Pol0_Constant8/1 -> scale_pol0_8/1
  scale_pol0_8/1 -> Pol0_Mux_Even/5
  Pol1_Constant8/1 -> scale_pol1_8/1
  scale_pol1_8/1 -> Pol1_Mux_Even/5
  Pol0_Constant10/1 -> scale_pol0_10/1
  scale_pol0_10/1 -> Pol0_Mux_Even/6
  Pol1_Constant10/1 -> scale_pol1_10/1
  scale_pol1_10/1 -> Pol1_Mux_Even/6
  Pol0_Constant12/1 -> scale_pol0_12/1
  scale_pol0_12/1 -> Pol0_Mux_Even/7
  Pol1_Constant12/1 -> scale_pol1_12/1
  scale_pol1_12/1 -> Pol1_Mux_Even/7
  Pol0_Constant14/1 -> scale_pol0_14/1
  scale_pol0_14/1 -> Pol0_Mux_Even/8
  Pol1_Constant14/1 -> scale_pol1_14/1
  scale_pol1_14/1 -> Pol1_Mux_Even/8
  Pol0_Constant16/1 -> scale_pol0_16/1
  scale_pol0_16/1 -> Pol0_Mux_Even/9
  Pol1_Constant16/1 -> scale_pol1_16/1
  scale_pol1_16/1 -> Pol1_Mux_Even/9

== system pasp_16i16c128s/pasp/scope_output1 ==
  rst : Inport  Port=1  LatchInput=off
  en : Inport  Port=2  LatchInput=off
  data_in : Inport  Port=3  LatchInput=off
  bram : xps_library/Shared BRAM  Tag=xps:bram  arith_type="Signed  (2's comp)"  addr_width=11  data_width=32  data_bin_pt=17  init_vals=[1:2^11]  sample_rate=1
  freeze_cntr : casper_library/Misc/freeze_cntr  CounterBits=11
  wires:
  freeze_cntr/1 -> bram/1
  freeze_cntr/2 -> bram/3
  en/1 -> freeze_cntr/1
  data_in/1 -> bram/2
  rst/1 -> freeze_cntr/2

== system pasp_16i16c128s/pasp/scope_output2 ==
  rst : Inport  Port=1  LatchInput=off
  en : Inport  Port=2  LatchInput=off
  data_in : Inport  Port=3  LatchInput=off
  bram : xps_library/Shared BRAM  Tag=xps:bram  arith_type="Signed  (2's comp)"  addr_width=11  data_width=32  data_bin_pt=17  init_vals=[1:2^11]  sample_rate=1
  freeze_cntr : casper_library/Misc/freeze_cntr  CounterBits=11
  wires:
  freeze_cntr/1 -> bram/1
  freeze_cntr/2 -> bram/3
  en/1 -> freeze_cntr/1
  data_in/1 -> bram/2
  rst/1 -> freeze_cntr/2

== system pasp_16i16c128s/pasp/scope_output3 ==
  rst : Inport  Port=1  LatchInput=off
  en : Inport  Port=2  LatchInput=off
  data_in : Inport  Port=3  LatchInput=off
  bram : xps_library/Shared BRAM  Tag=xps:bram  arith_type="Signed  (2's comp)"  addr_width=11  data_width=32  data_bin_pt=17  init_vals=[1:2^11]  sample_rate=1
  freeze_cntr : casper_library/Misc/freeze_cntr  CounterBits=11
  wires:
  rst/1 -> freeze_cntr/2
  data_in/1 -> bram/2
  en/1 -> freeze_cntr/1
  freeze_cntr/2 -> bram/3
  freeze_cntr/1 -> bram/1

== system pasp_16i16c128s/pasp/scope_output4 ==
  rst : Inport  Port=1  LatchInput=off
  en : Inport  Port=2  LatchInput=off
  data_in : Inport  Port=3  LatchInput=off
  bram : xps_library/Shared BRAM  Tag=xps:bram  arith_type="Signed  (2's comp)"  addr_width=11  data_width=32  data_bin_pt=17  init_vals=[1:2^11]  sample_rate=1
  freeze_cntr : casper_library/Misc/freeze_cntr  CounterBits=11
  wires:
  freeze_cntr/1 -> bram/1
  freeze_cntr/2 -> bram/3
  en/1 -> freeze_cntr/1
  data_in/1 -> bram/2
  rst/1 -> freeze_cntr/2

== system pasp_16i16c128s/pasp/scope_output5 ==
  rst : Inport  Port=1  LatchInput=off
  en : Inport  Port=2  LatchInput=off
  data_in : Inport  Port=3  LatchInput=off
  bram : xps_library/Shared BRAM  Tag=xps:bram  arith_type="Signed  (2's comp)"  addr_width=11  data_width=32  data_bin_pt=17  init_vals=[1:2^11]  sample_rate=1
  freeze_cntr : casper_library/Misc/freeze_cntr  CounterBits=11
  wires:
  freeze_cntr/1 -> bram/1
  freeze_cntr/2 -> bram/3
  en/1 -> freeze_cntr/1
  data_in/1 -> bram/2
  rst/1 -> freeze_cntr/2

== system pasp_16i16c128s/pasp/scope_output6 ==
  rst : Inport  Port=1  LatchInput=off
  en : Inport  Port=2  LatchInput=off
  data_in : Inport  Port=3  LatchInput=off
  bram : xps_library/Shared BRAM  Tag=xps:bram  arith_type="Signed  (2's comp)"  addr_width=11  data_width=32  data_bin_pt=17  init_vals=[1:2^11]  sample_rate=1
  freeze_cntr : casper_library/Misc/freeze_cntr  CounterBits=11
  wires:
  freeze_cntr/1 -> bram/1
  freeze_cntr/2 -> bram/3
  en/1 -> freeze_cntr/1
  data_in/1 -> bram/2
  rst/1 -> freeze_cntr/2

== system pasp_16i16c128s/pasp/scope_output7 ==
  rst : Inport  Port=1  LatchInput=off
  en : Inport  Port=2  LatchInput=off
  data_in : Inport  Port=3  LatchInput=off
  bram : xps_library/Shared BRAM  Tag=xps:bram  arith_type="Signed  (2's comp)"  addr_width=11  data_width=32  data_bin_pt=17  init_vals=[1:2^11]  sample_rate=1
  freeze_cntr : casper_library/Misc/freeze_cntr  CounterBits=11
  wires:
  rst/1 -> freeze_cntr/2
  data_in/1 -> bram/2
  en/1 -> freeze_cntr/1
  freeze_cntr/2 -> bram/3
  freeze_cntr/1 -> bram/1

== system pasp_16i16c128s/pasp/scope_output8 ==
  rst : Inport  Port=1  LatchInput=off
  en : Inport  Port=2  LatchInput=off
  data_in : Inport  Port=3  LatchInput=off
  bram : xps_library/Shared BRAM  Tag=xps:bram  arith_type="Signed  (2's comp)"  addr_width=11  data_width=32  data_bin_pt=17  init_vals=[1:2^11]  sample_rate=1
  freeze_cntr : casper_library/Misc/freeze_cntr  CounterBits=11
  wires:
  freeze_cntr/1 -> bram/1
  freeze_cntr/2 -> bram/3
  en/1 -> freeze_cntr/1
  data_in/1 -> bram/2
  rst/1 -> freeze_cntr/2

== system pasp_16i16c128s/pasp/sync_generator ==
  period : Inport  Port=1  LatchInput=off
  reset : Inport  Port=2  LatchInput=off
  Convert : xbsIndex_r3/Convert  arith_type=Boolean  n_bits=8  bin_pt=6  quantization=Truncate  overflow=Wrap  latency=1  explicit_period=off  period=1  dbl_ovrd=off  show_param=off  inserted_by_tool=off  pipeline=off
      settings: xl_area=[0, 0, 0, 0, 0, 0, 0]
  Counter : xbsIndex_r3/Counter  cnt_type=Free Running  n_bits=32  bin_pt=0  arith_type=Unsigned  start_count=1  cnt_to=Inf  cnt_by_val=1  operation=Up  explicit_period=on  period=1  load_pin=off  rst=on  en=off  dbl_ovrd=off  show_param=off  use_rpm=on  gen_core=off
      settings: xl_area=[0, 0, 0, 0, 0, 0, 0]
  Logical : xbsIndex_r3/Logical  logical_function=OR  inputs=2  precision=Full  arith_type=Unsigned  n_bits=8  bin_pt=2  align_bp=on  latency=0  explicit_period=off  period=1  en=off  dbl_ovrd=off  show_param=off
      settings: xl_area=[0, 0, 0, 0, 0, 0, 0]
  Relational : xbsIndex_r3/Relational  mode=a>=b  latency=1  explicit_period=off  period=1  en=off  dbl_ovrd=off  show_param=off
      settings: xl_area=[0, 0, 0, 0, 0, 0, 0]
  cns : xbsIndex_r3/Constant  const=4  equ=P=C  arith_type=Unsigned  n_bits=3  bin_pt=0  opselect=C  inp2=PCIN>>17  opr=+  inp1=P  carry=CIN  iostate=0  explicit_period=off  period=1  dbl_ovrd=off
  period_sub : xbsIndex_r3/AddSub  mode=Subtraction  precision=User Defined  arith_type=Unsigned  n_bits=32  bin_pt=0  quantization=Truncate  overflow=Wrap  latency=0  explicit_period=off  period=1  use_carryin=off  use_carryout=off  en=off  dbl_ovrd=off  show_param=off  use_core=on  pipeline=off  use_rpm=on  gen_core=off
      settings: xl_area=[0, 0, 0, 0, 0, 0, 0]
  posedge : casper_library/Misc/posedge  Tag=Rising Edge Detector
  sync : Outport
  wires:
  Counter/1 -> Relational/1
  Relational/1 -> Convert/1
  Convert/1 -> Logical/2
  Logical/1 -> Counter/1, posedge/1
  reset/1 -> Logical/1
  period/1 -> period_sub/1
  period_sub/1 -> Relational/2
  cns/1 -> period_sub/2
  posedge/1 -> sync/1
